simulink subsystem "PvtSubSys_VSM_LCK"  (R2020b)
settings: Solver=VariableStepAuto  StartTime=0.0  StopTime=10.0  RelTol=1e-3
values from neighbouring files (symbols this model uses):
  LCK_STATE : value not decoded    [LCK.sldd]
  P_VSM_LCK_A1 = 15.0    [LCK.sldd]
  P_VSM_LCK_AbsEspInTime = 3.0    [LCK.sldd]
  P_VSM_LCK_absLongitudeAccIn = 2.5    [LCK.sldd]
  P_VSM_LCK_absLongitudeAccOut = 3.0    [LCK.sldd]
  P_VSM_LCK_AccRateIn = 30.0    [LCK.sldd]
  P_VSM_LCK_AccRateInTime = 1.5    [LCK.sldd]
  P_VSM_LCK_AccRateOut = 80.0    [LCK.sldd]
  P_VSM_LCK_AccrPelOut = 30.0    [LCK.sldd]
  P_VSM_LCK_AccrPelRateOut = 0.0    [LCK.sldd]
  P_VSM_LCK_BrakePressIn = 3.0    [LCK.sldd]
  P_VSM_LCK_BrakePressInTime = 1.5    [LCK.sldd]
  P_VSM_LCK_BrakePressOut = 5.0    [LCK.sldd]
  P_VSM_LCK_C0 = 0.4    [LCK.sldd]
  P_VSM_LCK_DrvInputTrqValueIn = 2.0    [LCK.sldd]
  P_VSM_LCK_DrvInputTrqValueInTime = 3.0    [LCK.sldd]
  P_VSM_LCK_DrvInputTrqValueOut = 2.3    [LCK.sldd]
  P_VSM_LCK_dypreFactor = 1.0    [LCK.sldd]
  P_VSM_LCK_IdleInTime = 2.0    [LCK.sldd]
  P_VSM_LCK_LanechangeSwitch = 0.0    [LCK.sldd]
  P_VSM_LCK_LaneDouble = 1.0    [LCK.sldd]
  P_VSM_LCK_Lanewidthswitch = 1.0    [LCK.sldd]
  P_VSM_LCK_LateralAcceIn = 3.0    [LCK.sldd]
  P_VSM_LCK_LateralAcceInTime = 3.0    [LCK.sldd]
  P_VSM_LCK_LateralAcceOut = 3.5    [LCK.sldd]
  P_VSM_LCK_LCDrvInputTrqValueOut = 3.0    [LCK.sldd]
  P_VSM_LCK_LCOverrideTime = 0.6    [LCK.sldd]
  P_VSM_LCK_LCOverrideValue = 1.5    [LCK.sldd]
  P_VSM_LCK_LongitudeAccIn = 3.0    [LCK.sldd]
  P_VSM_LCK_LongitudeAccInTime = 3.0    [LCK.sldd]
  P_VSM_LCK_LongitudeAccOut = 3.5    [LCK.sldd]
  P_VSM_LCK_OverrideInTime = 3.0    [LCK.sldd]
  P_VSM_LCK_OverrideTime = 0.3    [LCK.sldd]
  P_VSM_LCK_OverrideValue = 1.2    [LCK.sldd]
  P_VSM_LCK_ParamA1 : value not decoded    [LCK.sldd]
  P_VSM_LCK_PreTime = 0.2    [LCK.sldd]
  P_VSM_LCK_State_Absesp_enable = 1.0    [LCK.sldd]
  P_VSM_LCK_State_Accpedalrate_enable = 0.0    [LCK.sldd]
  P_VSM_LCK_State_Breakpressure_enable = 1.0    [LCK.sldd]
  P_VSM_LCK_State_DriverInputTrqValue_enable = 1.0    [LCK.sldd]
  P_VSM_LCK_State_Eps_enable = 1.0    [LCK.sldd]
  P_VSM_LCK_State_ESSSts_enable = 1.0    [LCK.sldd]
  P_VSM_LCK_State_GEAR_enable = 1.0    [LCK.sldd]
  P_VSM_LCK_State_Handson_enable = 1.0    [LCK.sldd]
  P_VSM_LCK_State_IdleInTime_enable = 0.0    [LCK.sldd]
  P_VSM_LCK_State_Lane_enable = 1.0    [LCK.sldd]
  P_VSM_LCK_State_LaneChange_enable = 1.0    [LCK.sldd]
  P_VSM_LCK_State_LaneCurve_enable = 0.0    [LCK.sldd]
  P_VSM_LCK_State_LateralAcce_enable = 1.0    [LCK.sldd]
  P_VSM_LCK_State_LongitudeAcc_enable = 1.0    [LCK.sldd]
  P_VSM_LCK_State_LSMLine_enable = 1.0    [LCK.sldd]
  P_VSM_LCK_State_Overide_enable = 1.0    [LCK.sldd]
  P_VSM_LCK_State_Param_LaneCurve : value not decoded    [LCK.sldd]
  P_VSM_LCK_State_Param_LaneCurve_Offset : value not decoded    [LCK.sldd]
  P_VSM_LCK_State_Param_LaneWidth : value not decoded    [LCK.sldd]
  P_VSM_LCK_State_Param_LaneWidth_Offset : value not decoded    [LCK.sldd]
  P_VSM_LCK_State_SteerWheelAngle_enable = 1.0    [LCK.sldd]
  P_VSM_LCK_State_SteerWheelSpd_enable = 1.0    [LCK.sldd]
  P_VSM_LCK_State_TargetLaneIn_enable = 1.0    [LCK.sldd]
  P_VSM_LCK_State_TurnLight_enable = 1.0    [LCK.sldd]
  P_VSM_LCK_State_Vehspeed_enable = 1.0    [LCK.sldd]
  P_VSM_LCK_State_Yawsup_enable = 1.0    [LCK.sldd]
  P_VSM_LCK_SteerAngleSpdIn = 150.0    [LCK.sldd]
  P_VSM_LCK_SteerAngleSpdInTime = 3.0    [LCK.sldd]
  P_VSM_LCK_SteerAngleSpdOut = 200.0    [LCK.sldd]
  P_VSM_LCK_SteerWheelAngleIn = 70.0    [LCK.sldd]
  P_VSM_LCK_SteerWheelAngleInTime = 3.0    [LCK.sldd]
  P_VSM_LCK_SteerWheelAngleOut = 90.0    [LCK.sldd]
  P_VSM_LCK_T0 = 0.75    [LCK.sldd]
  P_VSM_LCK_T1 = 15.0    [LCK.sldd]
  P_VSM_LCK_TargetInSwitch = 0.0    [LCK.sldd]
  P_VSM_LCK_Warnarea1 = -0.55    [LCK.sldd]
  P_VSM_LCK_Warnarea2 = -0.35    [LCK.sldd]
  P_VSM_LCK_YawRateIn = 0.2    [LCK.sldd]
  P_VSM_LCK_YawRateInTime = 1.0    [LCK.sldd]
  P_VSM_LCK_YawRateOut = 0.25    [LCK.sldd]
undefined symbols (not defined in the file or in its folder): P_VSM_LSMC_SampleTime
libraries: simulink x275
(part 4 of 5)

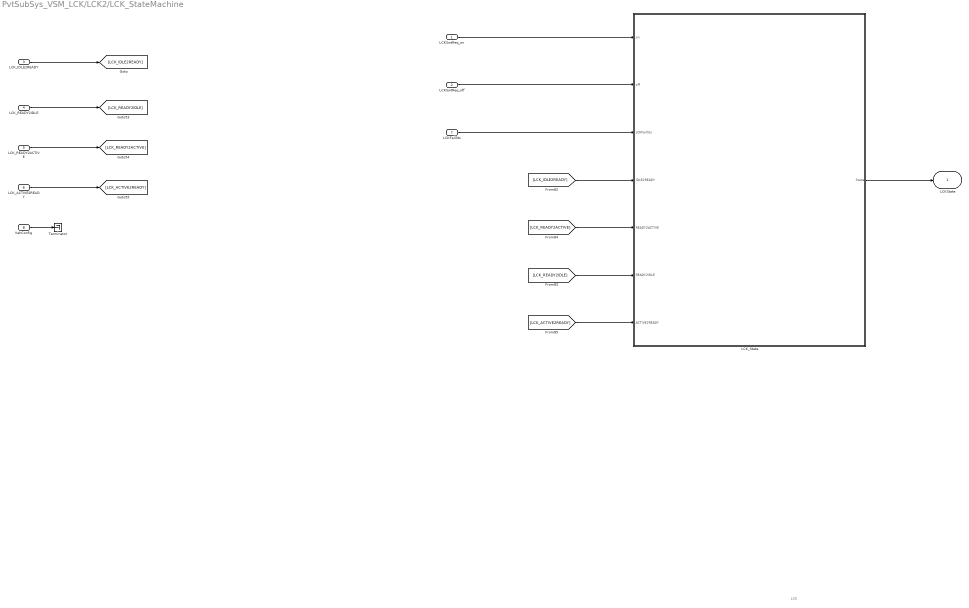
== system PvtSubSys_VSM_LCK/LCK2/LCK_StateMachine ==
  note: LCK
  LCKSwtReq_on : Inport
  LCKSwtReq_off : Inport  Port=2
  LCK_IDLE2READY : Inport  Port=3
  LCK_READY2IDLE : Inport  Port=4
  LCK_READY2ACTIVE : Inport  Port=5
  LCK_ACTIVE2READY : Inport  Port=6
  LCKFailSts : Inport  Port=7
  VehConfig : Inport  Port=8
  LCK_State : Stateflow chart  TreatAsAtomicUnit=on
  Terminator : Terminator
  LCKState : Outport
  wires:
  VehConfig/1 -> Terminator/1
  [LCK_READY2IDLE] -> LCK_State/6(READY2IDLE)
  LCKSwtReq_off/1 -> LCK_State/2(off)
  LCKSwtReq_on/1 -> LCK_State/1(on)
  LCK_ACTIVE2READY/1 -> [LCK_ACTIVE2READY]
  LCK_READY2ACTIVE/1 -> [LCK_READY2ACTIVE]
  LCK_READY2IDLE/1 -> [LCK_READY2IDLE]
  LCK_IDLE2READY/1 -> [LCK_IDLE2READY]
  [LCK_ACTIVE2READY] -> LCK_State/7(ACTIVE2READY)
  LCKFailSts/1 -> LCK_State/3(LCKFailSts)
  LCK_State/1(State) -> LCKState/1
  [LCK_IDLE2READY] -> LCK_State/4(IDLE2READY)
  [LCK_READY2ACTIVE] -> LCK_State/5(READY2ACTIVE)

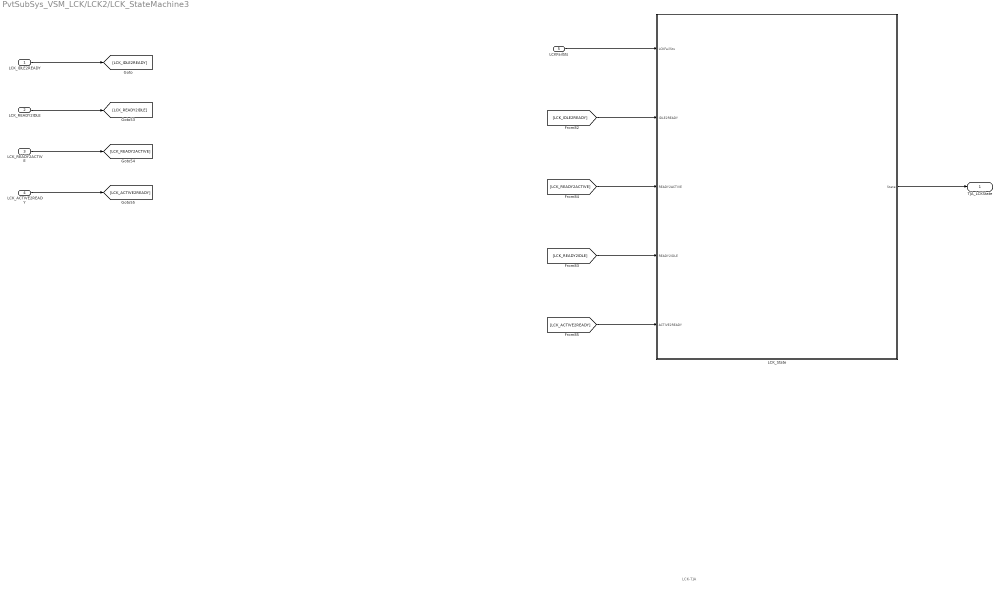
== system PvtSubSys_VSM_LCK/LCK2/LCK_StateMachine3 ==
  note: LCK-TJA
  LCK_IDLE2READY : Inport
  LCK_READY2IDLE : Inport  Port=2
  LCK_READY2ACTIVE : Inport  Port=3
  LCK_ACTIVE2READY : Inport  Port=4
  LCKFailSts : Inport  Port=5
  LCK_State : Stateflow chart  TreatAsAtomicUnit=on
  TJA_LCKState : Outport
  wires:
  [LCK_READY2IDLE] -> LCK_State/4(READY2IDLE)
  LCK_ACTIVE2READY/1 -> [LCK_ACTIVE2READY]
  LCK_READY2ACTIVE/1 -> [LCK_READY2ACTIVE]
  LCK_READY2IDLE/1 -> [LCK_READY2IDLE]
  LCK_IDLE2READY/1 -> [LCK_IDLE2READY]
  [LCK_ACTIVE2READY] -> LCK_State/5(ACTIVE2READY)
  LCKFailSts/1 -> LCK_State/1(LCKFailSts)
  LCK_State/1(State) -> TJA_LCKState/1
  [LCK_IDLE2READY] -> LCK_State/2(IDLE2READY)
  [LCK_READY2ACTIVE] -> LCK_State/3(READY2ACTIVE)

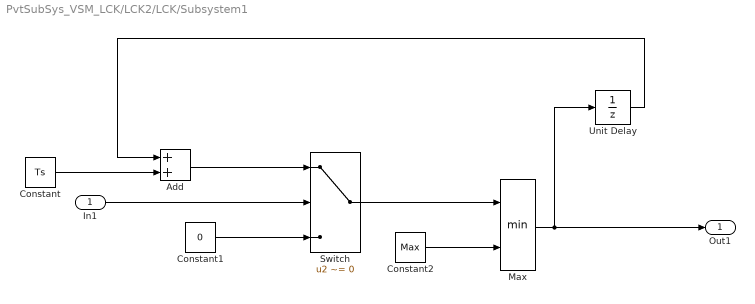
== system PvtSubSys_VSM_LCK/LCK2/LCK/Subsystem1 ==
  In1 : Inport
  Add : Sum
  Constant : Constant  Value=Ts
  Constant1 : Constant  Value=0
  Constant2 : Constant  Value=Max
  Max : MinMax  Inputs=2
  Switch : Switch  Criteria=u2 ~= 0
  Unit Delay : UnitDelay  SampleTime=-1  HasFrameUpgradeWarning=on
  Out1 : Outport
  wires:
  Switch/1 -> Max/1
  Constant2/1 -> Max/2
  Max/1 -> Out1/1, Unit Delay/1
  Add/1 -> Switch/1
  Constant1/1 -> Switch/3
  Constant/1 -> Add/2
  In1/1 -> Switch/2
  Unit Delay/1 -> Add/1

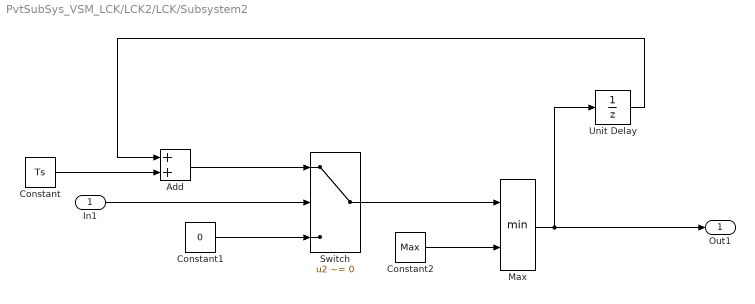
== system PvtSubSys_VSM_LCK/LCK2/LCK/Subsystem2 ==
  In1 : Inport
  Add : Sum
  Constant : Constant  Value=Ts
  Constant1 : Constant  Value=0
  Constant2 : Constant  Value=Max
  Max : MinMax  Inputs=2
  Switch : Switch  Criteria=u2 ~= 0
  Unit Delay : UnitDelay  SampleTime=-1  HasFrameUpgradeWarning=on
  Out1 : Outport
  wires:
  Unit Delay/1 -> Add/1
  In1/1 -> Switch/2
  Constant/1 -> Add/2
  Constant1/1 -> Switch/3
  Add/1 -> Switch/1
  Max/1 -> Unit Delay/1, Out1/1
  Constant2/1 -> Max/2
  Switch/1 -> Max/1

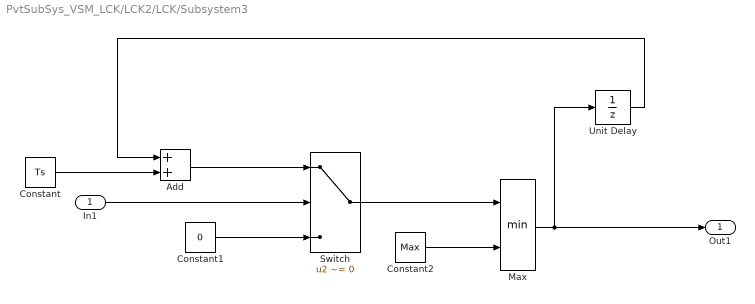
== system PvtSubSys_VSM_LCK/LCK2/LCK/Subsystem3 ==
  In1 : Inport
  Add : Sum
  Constant : Constant  Value=Ts
  Constant1 : Constant  Value=0
  Constant2 : Constant  Value=Max
  Max : MinMax  Inputs=2
  Switch : Switch  Criteria=u2 ~= 0
  Unit Delay : UnitDelay  SampleTime=-1  HasFrameUpgradeWarning=on
  Out1 : Outport
  wires:
  Switch/1 -> Max/1
  Constant2/1 -> Max/2
  Max/1 -> Out1/1, Unit Delay/1
  Add/1 -> Switch/1
  Constant1/1 -> Switch/3
  Constant/1 -> Add/2
  In1/1 -> Switch/2
  Unit Delay/1 -> Add/1

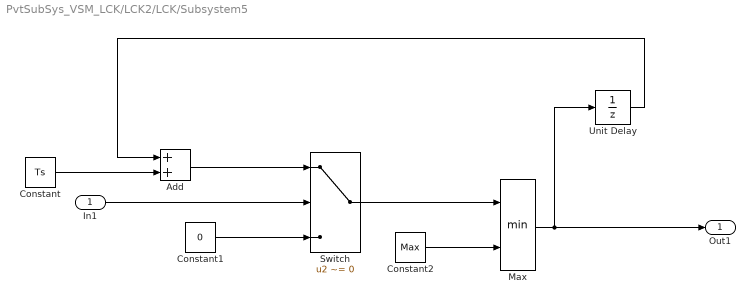
== system PvtSubSys_VSM_LCK/LCK2/LCK/Subsystem5 ==
  In1 : Inport
  Add : Sum
  Constant : Constant  Value=Ts
  Constant1 : Constant  Value=0
  Constant2 : Constant  Value=Max
  Max : MinMax  Inputs=2
  Switch : Switch  Criteria=u2 ~= 0
  Unit Delay : UnitDelay  SampleTime=-1  HasFrameUpgradeWarning=on
  Out1 : Outport
  wires:
  Unit Delay/1 -> Add/1
  In1/1 -> Switch/2
  Constant/1 -> Add/2
  Constant1/1 -> Switch/3
  Add/1 -> Switch/1
  Max/1 -> Unit Delay/1, Out1/1
  Constant2/1 -> Max/2
  Switch/1 -> Max/1

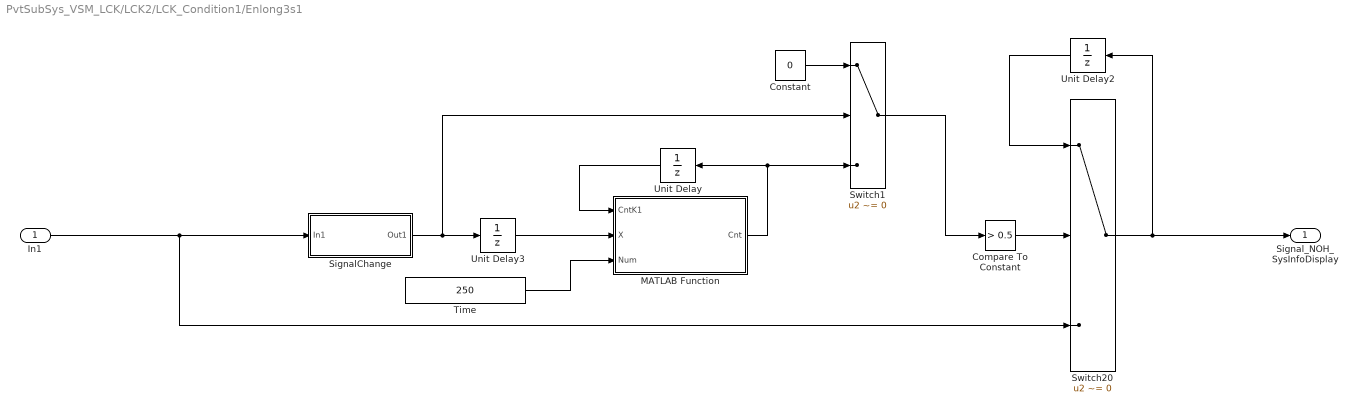
== system PvtSubSys_VSM_LCK/LCK2/LCK_Condition1/Enlong3s1 ==
  In1 : Inport
  Compare To Constant : simulink/Logic and Bit Operations/Compare To Constant  relop=>  const=0.5  OutDataTypeStr=boolean
  Constant : Constant  Value=0  OutDataTypeStr=uint16
  MATLAB Function : MATLAB Function  TreatAsAtomicUnit=on
  SignalChange : Subsystem
  Switch1 : Switch  Criteria=u2 ~= 0
  Switch20 : Switch  Criteria=u2 ~= 0
  Time : Constant  Value=250  OutDataTypeStr=uint16
  Unit Delay : UnitDelay  SampleTime=-1  HasFrameUpgradeWarning=on
  Unit Delay2 : UnitDelay  SampleTime=-1  HasFrameUpgradeWarning=on
  Unit Delay3 : UnitDelay  SampleTime=-1  HasFrameUpgradeWarning=on
  Signal_NOH_SysInfoDisplay : Outport
  wires:
  Time/1 -> MATLAB Function/3(Num)
  Switch20/1 -> Signal_NOH_SysInfoDisplay/1, Unit Delay2/1
  Unit Delay2/1 -> Switch20/1
  Unit Delay3/1 -> MATLAB Function/2(X)
  Compare To Constant/1 -> Switch20/2
  Switch1/1 -> Compare To Constant/1
  MATLAB Function/1(Cnt) -> Unit Delay/1, Switch1/3
  Constant/1 -> Switch1/1
  Unit Delay/1 -> MATLAB Function/1(CntK1)
  SignalChange/1(Out1) -> Unit Delay3/1, Switch1/2
  In1/1 -> SignalChange/1(In1), Switch20/3

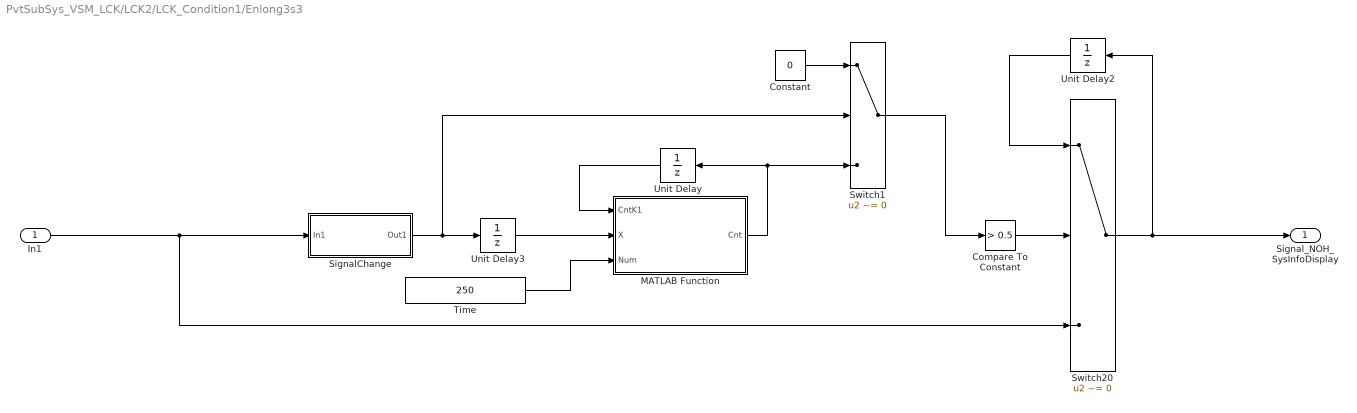
== system PvtSubSys_VSM_LCK/LCK2/LCK_Condition1/Enlong3s3 ==
  In1 : Inport
  Compare To Constant : simulink/Logic and Bit Operations/Compare To Constant  relop=>  const=0.5  OutDataTypeStr=boolean
  Constant : Constant  Value=0  OutDataTypeStr=uint16
  MATLAB Function : MATLAB Function  TreatAsAtomicUnit=on
  SignalChange : Subsystem
  Switch1 : Switch  Criteria=u2 ~= 0
  Switch20 : Switch  Criteria=u2 ~= 0
  Time : Constant  Value=250  OutDataTypeStr=uint16
  Unit Delay : UnitDelay  SampleTime=-1  HasFrameUpgradeWarning=on
  Unit Delay2 : UnitDelay  SampleTime=-1  HasFrameUpgradeWarning=on
  Unit Delay3 : UnitDelay  SampleTime=-1  HasFrameUpgradeWarning=on
  Signal_NOH_SysInfoDisplay : Outport
  wires:
  In1/1 -> Switch20/3, SignalChange/1(In1)
  SignalChange/1(Out1) -> Switch1/2, Unit Delay3/1
  Unit Delay/1 -> MATLAB Function/1(CntK1)
  Constant/1 -> Switch1/1
  MATLAB Function/1(Cnt) -> Switch1/3, Unit Delay/1
  Switch1/1 -> Compare To Constant/1
  Compare To Constant/1 -> Switch20/2
  Unit Delay3/1 -> MATLAB Function/2(X)
  Unit Delay2/1 -> Switch20/1
  Switch20/1 -> Unit Delay2/1, Signal_NOH_SysInfoDisplay/1
  Time/1 -> MATLAB Function/3(Num)

== system PvtSubSys_VSM_LCK/LCK2/LCK_Condition1/Subsystem1 ==
  In1 : Inport
  Add : Sum
  Constant : Constant  Value=Ts
  Constant1 : Constant  Value=0
  Constant2 : Constant  Value=Max
  Max : MinMax  Inputs=2
  Switch : Switch  Criteria=u2 ~= 0
  Unit Delay : UnitDelay  SampleTime=-1  HasFrameUpgradeWarning=on
  Out1 : Outport
  wires:
  Switch/1 -> Max/1
  Constant2/1 -> Max/2
  Max/1 -> Out1/1, Unit Delay/1
  Add/1 -> Switch/1
  Constant1/1 -> Switch/3
  Constant/1 -> Add/2
  In1/1 -> Switch/2
  Unit Delay/1 -> Add/1

== system PvtSubSys_VSM_LCK/LCK2/LCK_Condition1/Subsystem10 ==
  In1 : Inport
  Add : Sum
  Constant : Constant  Value=Ts
  Constant1 : Constant  Value=0
  Constant2 : Constant  Value=Max
  Max : MinMax  Inputs=2
  Switch : Switch  Criteria=u2 ~= 0
  Unit Delay : UnitDelay  SampleTime=-1  HasFrameUpgradeWarning=on
  Out1 : Outport
  wires:
  Unit Delay/1 -> Add/1
  In1/1 -> Switch/2
  Constant/1 -> Add/2
  Constant1/1 -> Switch/3
  Add/1 -> Switch/1
  Max/1 -> Unit Delay/1, Out1/1
  Constant2/1 -> Max/2
  Switch/1 -> Max/1

== system PvtSubSys_VSM_LCK/LCK2/LCK_Condition1/Subsystem11 ==
  In1 : Inport
  Add : Sum
  Constant : Constant  Value=Ts
  Constant1 : Constant  Value=0
  Constant2 : Constant  Value=Max
  Max : MinMax  Inputs=2
  Switch : Switch  Criteria=u2 ~= 0
  Unit Delay : UnitDelay  SampleTime=-1  HasFrameUpgradeWarning=on
  Out1 : Outport
  wires:
  Switch/1 -> Max/1
  Constant2/1 -> Max/2
  Max/1 -> Out1/1, Unit Delay/1
  Add/1 -> Switch/1
  Constant1/1 -> Switch/3
  Constant/1 -> Add/2
  In1/1 -> Switch/2
  Unit Delay/1 -> Add/1

== system PvtSubSys_VSM_LCK/LCK2/LCK_Condition1/Subsystem12 ==
  In1 : Inport
  Add : Sum
  Constant : Constant  Value=Ts
  Constant1 : Constant  Value=0
  Constant2 : Constant  Value=Max
  Max : MinMax  Inputs=2
  Switch : Switch  Criteria=u2 ~= 0
  Unit Delay : UnitDelay  SampleTime=-1  HasFrameUpgradeWarning=on
  Out1 : Outport
  wires:
  Unit Delay/1 -> Add/1
  In1/1 -> Switch/2
  Constant/1 -> Add/2
  Constant1/1 -> Switch/3
  Add/1 -> Switch/1
  Max/1 -> Unit Delay/1, Out1/1
  Constant2/1 -> Max/2
  Switch/1 -> Max/1

== system PvtSubSys_VSM_LCK/LCK2/LCK_Condition1/Subsystem13 ==
  In1 : Inport
  Add : Sum
  Constant : Constant  Value=Ts
  Constant1 : Constant  Value=0
  Constant2 : Constant  Value=Max
  Max : MinMax  Inputs=2
  Switch : Switch  Criteria=u2 ~= 0
  Unit Delay : UnitDelay  SampleTime=-1  HasFrameUpgradeWarning=on
  Out1 : Outport
  wires:
  Switch/1 -> Max/1
  Constant2/1 -> Max/2
  Max/1 -> Out1/1, Unit Delay/1
  Add/1 -> Switch/1
  Constant1/1 -> Switch/3
  Constant/1 -> Add/2
  In1/1 -> Switch/2
  Unit Delay/1 -> Add/1

== system PvtSubSys_VSM_LCK/LCK2/LCK_Condition1/Subsystem14 ==
  In1 : Inport
  Add : Sum
  Constant : Constant  Value=Ts
  Constant1 : Constant  Value=0
  Constant2 : Constant  Value=Max
  Max : MinMax  Inputs=2
  Switch : Switch  Criteria=u2 ~= 0
  Unit Delay : UnitDelay  SampleTime=-1  HasFrameUpgradeWarning=on
  Out1 : Outport
  wires:
  Unit Delay/1 -> Add/1
  In1/1 -> Switch/2
  Constant/1 -> Add/2
  Constant1/1 -> Switch/3
  Add/1 -> Switch/1
  Max/1 -> Unit Delay/1, Out1/1
  Constant2/1 -> Max/2
  Switch/1 -> Max/1

== system PvtSubSys_VSM_LCK/LCK2/LCK_Condition1/Subsystem15 ==
  In1 : Inport
  Add : Sum
  Constant : Constant  Value=Ts
  Constant1 : Constant  Value=0
  Constant2 : Constant  Value=Max
  Max : MinMax  Inputs=2
  Switch : Switch  Criteria=u2 ~= 0
  Unit Delay : UnitDelay  SampleTime=-1  HasFrameUpgradeWarning=on
  Out1 : Outport
  wires:
  Switch/1 -> Max/1
  Constant2/1 -> Max/2
  Max/1 -> Out1/1, Unit Delay/1
  Add/1 -> Switch/1
  Constant1/1 -> Switch/3
  Constant/1 -> Add/2
  In1/1 -> Switch/2
  Unit Delay/1 -> Add/1

== system PvtSubSys_VSM_LCK/LCK2/LCK_Condition1/Subsystem16 ==
  In1 : Inport
  Add : Sum
  Constant : Constant  Value=Ts
  Constant1 : Constant  Value=0
  Constant2 : Constant  Value=Max
  Max : MinMax  Inputs=2
  Switch : Switch  Criteria=u2 ~= 0
  Unit Delay : UnitDelay  SampleTime=-1  HasFrameUpgradeWarning=on
  Out1 : Outport
  wires:
  Unit Delay/1 -> Add/1
  In1/1 -> Switch/2
  Constant/1 -> Add/2
  Constant1/1 -> Switch/3
  Add/1 -> Switch/1
  Max/1 -> Unit Delay/1, Out1/1
  Constant2/1 -> Max/2
  Switch/1 -> Max/1

== system PvtSubSys_VSM_LCK/LCK2/LCK_Condition1/Subsystem17 ==
  In1 : Inport
  Add : Sum
  Constant : Constant  Value=Ts
  Constant1 : Constant  Value=0
  Constant2 : Constant  Value=Max
  Max : MinMax  Inputs=2
  Switch : Switch  Criteria=u2 ~= 0
  Unit Delay : UnitDelay  SampleTime=-1  HasFrameUpgradeWarning=on
  Out1 : Outport
  wires:
  Unit Delay/1 -> Add/1
  In1/1 -> Switch/2
  Constant/1 -> Add/2
  Constant1/1 -> Switch/3
  Add/1 -> Switch/1
  Max/1 -> Unit Delay/1, Out1/1
  Constant2/1 -> Max/2
  Switch/1 -> Max/1

== system PvtSubSys_VSM_LCK/LCK2/LCK_Condition1/Subsystem18 ==
  In1 : Inport
  Add : Sum
  Constant : Constant  Value=Ts
  Constant1 : Constant  Value=0
  Constant2 : Constant  Value=Max
  Max : MinMax  Inputs=2
  Switch : Switch  Criteria=u2 ~= 0
  Unit Delay : UnitDelay  SampleTime=-1  HasFrameUpgradeWarning=on
  Out1 : Outport
  wires:
  Unit Delay/1 -> Add/1
  In1/1 -> Switch/2
  Constant/1 -> Add/2
  Constant1/1 -> Switch/3
  Add/1 -> Switch/1
  Max/1 -> Unit Delay/1, Out1/1
  Constant2/1 -> Max/2
  Switch/1 -> Max/1

== system PvtSubSys_VSM_LCK/LCK2/LCK_Condition1/Subsystem19 ==
  In1 : Inport
  Add : Sum
  Constant : Constant  Value=Ts
  Constant1 : Constant  Value=0
  Constant2 : Constant  Value=Max
  Max : MinMax  Inputs=2
  Switch : Switch  Criteria=u2 ~= 0
  Unit Delay : UnitDelay  SampleTime=-1  HasFrameUpgradeWarning=on
  Out1 : Outport
  wires:
  Switch/1 -> Max/1
  Constant2/1 -> Max/2
  Max/1 -> Out1/1, Unit Delay/1
  Add/1 -> Switch/1
  Constant1/1 -> Switch/3
  Constant/1 -> Add/2
  In1/1 -> Switch/2
  Unit Delay/1 -> Add/1

== system PvtSubSys_VSM_LCK/LCK2/LCK_Condition1/Subsystem2 ==
  In1 : Inport
  Add : Sum
  Constant : Constant  Value=Ts
  Constant1 : Constant  Value=0
  Constant2 : Constant  Value=Max
  Max : MinMax  Inputs=2
  Switch : Switch  Criteria=u2 ~= 0
  Unit Delay : UnitDelay  SampleTime=-1  HasFrameUpgradeWarning=on
  Out1 : Outport
  wires:
  Unit Delay/1 -> Add/1
  In1/1 -> Switch/2
  Constant/1 -> Add/2
  Constant1/1 -> Switch/3
  Add/1 -> Switch/1
  Max/1 -> Unit Delay/1, Out1/1
  Constant2/1 -> Max/2
  Switch/1 -> Max/1

== system PvtSubSys_VSM_LCK/LCK2/LCK_Condition1/Subsystem20 ==
  In1 : Inport
  Add : Sum
  Constant : Constant  Value=Ts
  Constant1 : Constant  Value=0
  Constant2 : Constant  Value=Max
  Max : MinMax  Inputs=2
  Switch : Switch  Criteria=u2 ~= 0
  Unit Delay : UnitDelay  SampleTime=-1  HasFrameUpgradeWarning=on
  Out1 : Outport
  wires:
  Switch/1 -> Max/1
  Constant2/1 -> Max/2
  Max/1 -> Out1/1, Unit Delay/1
  Add/1 -> Switch/1
  Constant1/1 -> Switch/3
  Constant/1 -> Add/2
  In1/1 -> Switch/2
  Unit Delay/1 -> Add/1

== system PvtSubSys_VSM_LCK/LCK2/LCK_Condition1/Subsystem21 ==
  In1 : Inport
  Add : Sum
  Constant : Constant  Value=Ts
  Constant1 : Constant  Value=0
  Constant2 : Constant  Value=Max
  Max : MinMax  Inputs=2
  Switch : Switch  Criteria=u2 ~= 0
  Unit Delay : UnitDelay  SampleTime=-1  HasFrameUpgradeWarning=on
  Out1 : Outport
  wires:
  Switch/1 -> Max/1
  Constant2/1 -> Max/2
  Max/1 -> Out1/1, Unit Delay/1
  Add/1 -> Switch/1
  Constant1/1 -> Switch/3
  Constant/1 -> Add/2
  In1/1 -> Switch/2
  Unit Delay/1 -> Add/1

== system PvtSubSys_VSM_LCK/LCK2/LCK_Condition1/Subsystem3 ==
  In1 : Inport
  Add : Sum
  Constant : Constant  Value=Ts
  Constant1 : Constant  Value=0
  Constant2 : Constant  Value=Max
  Max : MinMax  Inputs=2
  Switch : Switch  Criteria=u2 ~= 0
  Unit Delay : UnitDelay  SampleTime=-1  HasFrameUpgradeWarning=on
  Out1 : Outport
  wires:
  Unit Delay/1 -> Add/1
  In1/1 -> Switch/2
  Constant/1 -> Add/2
  Constant1/1 -> Switch/3
  Add/1 -> Switch/1
  Max/1 -> Unit Delay/1, Out1/1
  Constant2/1 -> Max/2
  Switch/1 -> Max/1

== system PvtSubSys_VSM_LCK/LCK2/LCK_Condition1/Subsystem4 ==
  In1 : Inport
  Add : Sum
  Constant : Constant  Value=Ts
  Constant1 : Constant  Value=0
  Constant2 : Constant  Value=Max
  Max : MinMax  Inputs=2
  Switch : Switch  Criteria=u2 ~= 0
  Unit Delay : UnitDelay  SampleTime=-1  HasFrameUpgradeWarning=on
  Out1 : Outport
  wires:
  Unit Delay/1 -> Add/1
  In1/1 -> Switch/2
  Constant/1 -> Add/2
  Constant1/1 -> Switch/3
  Add/1 -> Switch/1
  Max/1 -> Unit Delay/1, Out1/1
  Constant2/1 -> Max/2
  Switch/1 -> Max/1

== system PvtSubSys_VSM_LCK/LCK2/LCK_Condition1/Subsystem5 ==
  In1 : Inport
  Add : Sum
  Constant : Constant  Value=Ts
  Constant1 : Constant  Value=0
  Constant2 : Constant  Value=Max
  Max : MinMax  Inputs=2
  Switch : Switch  Criteria=u2 ~= 0
  Unit Delay : UnitDelay  SampleTime=-1  HasFrameUpgradeWarning=on
  Out1 : Outport
  wires:
  Switch/1 -> Max/1
  Constant2/1 -> Max/2
  Max/1 -> Out1/1, Unit Delay/1
  Add/1 -> Switch/1
  Constant1/1 -> Switch/3
  Constant/1 -> Add/2
  In1/1 -> Switch/2
  Unit Delay/1 -> Add/1

== system PvtSubSys_VSM_LCK/LCK2/LCK_Condition1/Subsystem7 ==
  In1 : Inport
  Add : Sum
  Constant : Constant  Value=Ts
  Constant1 : Constant  Value=0
  Constant2 : Constant  Value=Max
  Max : MinMax  Inputs=2
  Switch : Switch  Criteria=u2 ~= 0
  Unit Delay : UnitDelay  SampleTime=-1  HasFrameUpgradeWarning=on
  Out1 : Outport
  wires:
  Switch/1 -> Max/1
  Constant2/1 -> Max/2
  Max/1 -> Out1/1, Unit Delay/1
  Add/1 -> Switch/1
  Constant1/1 -> Switch/3
  Constant/1 -> Add/2
  In1/1 -> Switch/2
  Unit Delay/1 -> Add/1

== system PvtSubSys_VSM_LCK/LCK2/LCK_Condition1/Subsystem8 ==
  In1 : Inport
  Add : Sum
  Constant : Constant  Value=Ts
  Constant1 : Constant  Value=0
  Constant2 : Constant  Value=Max
  Max : MinMax  Inputs=2
  Switch : Switch  Criteria=u2 ~= 0
  Unit Delay : UnitDelay  SampleTime=-1  HasFrameUpgradeWarning=on
  Out1 : Outport
  wires:
  Switch/1 -> Max/1
  Constant2/1 -> Max/2
  Max/1 -> Out1/1, Unit Delay/1
  Add/1 -> Switch/1
  Constant1/1 -> Switch/3
  Constant/1 -> Add/2
  In1/1 -> Switch/2
  Unit Delay/1 -> Add/1

== system PvtSubSys_VSM_LCK/LCK2/LCK_Condition1/Subsystem9 ==
  In1 : Inport
  Add : Sum
  Constant : Constant  Value=Ts
  Constant1 : Constant  Value=0
  Constant2 : Constant  Value=Max
  Max : MinMax  Inputs=2
  Switch : Switch  Criteria=u2 ~= 0
  Unit Delay : UnitDelay  SampleTime=-1  HasFrameUpgradeWarning=on
  Out1 : Outport
  wires:
  Unit Delay/1 -> Add/1
  In1/1 -> Switch/2
  Constant/1 -> Add/2
  Constant1/1 -> Switch/3
  Add/1 -> Switch/1
  Max/1 -> Unit Delay/1, Out1/1
  Constant2/1 -> Max/2
  Switch/1 -> Max/1

== system PvtSubSys_VSM_LCK/LCK2/LCK_Condition1/Enlong3s1/SignalChange ==
  In1 : Inport
  Compare To Constant1 : simulink/Logic and Bit Operations/Compare To Constant  relop=~=  const=0  OutDataTypeStr=boolean
  Detect Decrease : simulink/Logic and Bit Operations/Detect Decrease  vinit=0.0  OutDataTypeStr=boolean
  Detect Increase3 : simulink/Logic and Bit Operations/Detect Increase  vinit=0.0  OutDataTypeStr=boolean
  Logical Operator : Logic  Operator=OR  AllPortsSameDT=off  OutDataTypeStr=boolean
  Logical Operator1 : Logic  AllPortsSameDT=off  OutDataTypeStr=boolean
  Out1 : Outport
  wires:
  Detect Decrease/1 -> Logical Operator/1
  Logical Operator/1 -> Logical Operator1/2
  Logical Operator1/1 -> Out1/1
  Compare To Constant1/1 -> Logical Operator1/1
  Detect Increase3/1 -> Logical Operator/2
  In1/1 -> Compare To Constant1/1, Detect Decrease/1, Detect Increase3/1

== system PvtSubSys_VSM_LCK/LCK2/LCK_Condition1/Enlong3s3/SignalChange ==
  In1 : Inport
  Compare To Constant1 : simulink/Logic and Bit Operations/Compare To Constant  relop=~=  const=0  OutDataTypeStr=boolean
  Detect Decrease : simulink/Logic and Bit Operations/Detect Decrease  vinit=0.0  OutDataTypeStr=boolean
  Detect Increase3 : simulink/Logic and Bit Operations/Detect Increase  vinit=0.0  OutDataTypeStr=boolean
  Logical Operator : Logic  Operator=OR  AllPortsSameDT=off  OutDataTypeStr=boolean
  Logical Operator1 : Logic  AllPortsSameDT=off  OutDataTypeStr=boolean
  Out1 : Outport
  wires:
  In1/1 -> Detect Increase3/1, Detect Decrease/1, Compare To Constant1/1
  Detect Increase3/1 -> Logical Operator/2
  Compare To Constant1/1 -> Logical Operator1/1
  Logical Operator1/1 -> Out1/1
  Logical Operator/1 -> Logical Operator1/2
  Detect Decrease/1 -> Logical Operator/1

== matlab function PvtSubSys_VSM_LCK/LCK2/LCK/MATLAB Function2 ==
  data: OutCount input single size=1; InCount input single size=1; LCK_LeftWarn input boolean size=1; LCKWarning output uint8 size=1; LCK_RightWarn input boolean size=1; LCKState input uint8 size=1; LCKWarningK1 input uint8 size=1
function LCKWarning = fcn(OutCount, InCount, LCK_LeftWarn, LCK_RightWarn, LCKState, LCKWarningK1)
LCKWarning=uint8(0);
if LCKWarningK1==uint8(3)       %default状态
    if LCK_LeftWarn==uint8(1) && LCKState==uint8(3) && InCount>single(150) %抑制3s
        LCKWarning=uint8(1);
    elseif LCK_RightWarn==uint8(1) && LCKState==uint8(3) && InCount>single(150)
        LCKWarning=uint8(2);
    elseif LCK_LeftWarn==uint8(0) && LCK_RightWarn==uint8(0)
        LCKWarning=uint8(0);
    else
        LCKWarning=uint8(3);
    end
elseif  LCKWarningK1==uint8(1) || LCKWarningK1==uint8(2)   %非default状态
    if LCK_LeftWarn==uint8(1) && LCK_RightWarn==uint8(0) && LCKState==uint8(3)
        if OutCount<single(200)  %4s后抑制
            LCKWarning=uint8(1);
        else
            LCKWarning=uint8(3);
        end
    elseif LCK_LeftWarn==uint8(0) && LCK_RightWarn==uint8(1) && LCKState==uint8(3)
        if OutCount<single(200)
            LCKWarning=uint8(2);
        else
            LCKWarning=uint8(3);
        end
        
    elseif LCK_LeftWarn==uint8(0) && LCK_RightWarn==uint8(0)
        LCKWarning=uint8(0);
    end
elseif  LCKWarningK1==uint8(0)
    if LCK_LeftWarn==uint8(1) && LCK_RightWarn==uint8(0) && LCKState==uint8(3)
        LCKWarning=uint8(1);
    elseif LCK_LeftWarn==uint8(0) && LCK_RightWarn==uint8(1) && LCKState==uint8(3)
        LCKWarning=uint8(2);
    end
end

== matlab function PvtSubSys_VSM_LCK/LCK2/LCK/MATLAB Function3 ==
  data: data input single size=1; LCKWarning input uint8 size=1; OutCount output single size=1; InCount output single size=1; data1 input single size=1
function [OutCount,InCount] = fcn(data, LCKWarning, data1)
OutCount=single(0);
 InCount=single(0);
if LCKWarning==uint8(1) || LCKWarning==uint8(2)
    OutCount=data+1;  
elseif LCKWarning==uint8(3)
    InCount=data1+1;
end

== matlab function PvtSubSys_VSM_LCK/LCK2/LCK_Condition1/MATLAB Function ==
  data: LeftChangefg input; y output; RightChangefg input; Ldy input; Rdy input; Lfgk1 input; Lfg output; Rfgk1 input; Rfg output
function [y,Lfg,Rfg] = fcn(LeftChangefg,RightChangefg,Ldy,Rdy,Lfgk1,Rfgk1)
y=1;
Lfg=0;
Rfg=0;
if LeftChangefg>0
    Lfg=1;
    y=0;
elseif Lfgk1>0
    Lfg=1;
    y=0;
    if Rdy>0
        Lfg=0;
        y=1;
    end
    
end

if RightChangefg>0
    Rfg=1;
    y=0;
elseif Rfgk1>0
    Rfg=1;
    y=0;
    if Ldy>0
        Rfg=0;
        y=1;
    end
    
end

== matlab function PvtSubSys_VSM_LCK/LCK2/LCK_Condition1/MATLAB Function3 ==
  data: Ready2Idle input; Ready2IdleK1 input; LCKSts input; CountK1 input; Count output
function Count= fcn(Ready2Idle,Ready2IdleK1,LCKSts,CountK1)
Count=0;
if LCKSts==1
    if Ready2Idle==1 || Ready2IdleK1==1
        Count=CountK1+1;
    elseif CountK1>0 && Ready2Idle==0
        Count=CountK1+1;
    end
elseif LCKSts==2 || LCKSts==3 
    Count=0;
elseif LCKSts==0 || LCKSts==7
    Count=9999;
end

== stateflow chart PvtSubSys_VSM_LCK/LCK2/LCK_StateMachine/LCK_State ==
  state MAINST_ERROR
    en:State=LCK_STATE.LCK_Error;
  state MAINST_OFF
    en:State=LCK_STATE.LCK_Off;
  state MAINST_ON
    state SUBST_IDLE
      en: State=LCK_STATE.LCK_Idle;
    state enabled
      state SUBST_READY
        en:State=LCK_STATE.LCK_Ready;
      state SUBST_ACTIVE
        en:State=LCK_STATE.LCK_Active;
      (default) -> (junction 367)
      (junction 367) -> SUBST_READY [order 2]
      (junction 367) -> SUBST_ACTIVE [order 1] : [READY2ACTIVE]
      SUBST_READY -> SUBST_ACTIVE : [READY2ACTIVE]
      SUBST_ACTIVE -> SUBST_READY : [ACTIVE2READY]
    (junction 366) -> SUBST_IDLE [order 2]
    SUBST_IDLE -> enabled : [IDLE2READY]
    enabled -> SUBST_IDLE : [READY2IDLE]
    (default) -> (junction 366)
    (junction 366) -> enabled [order 1] : [IDLE2READY]
  (default) -> MAINST_OFF
  MAINST_OFF -> MAINST_ERROR [order 1] : [LCKFailSts==1 && on ]
  MAINST_ERROR -> MAINST_OFF [order 1] : [off]
  MAINST_OFF -> MAINST_ON [order 2] : [on]
  MAINST_ON -> MAINST_OFF [order 1] : [off]
  MAINST_ON -> MAINST_ERROR [order 2] : [LCKFailSts==1]
  MAINST_ERROR -> MAINST_ON [order 2] : [LCKFailSts==0]
  data: on input; off input; LCKFailSts input; State output Enum: LCK_STATE =LCK_STATE.LCK_Off;; IDLE2READY input; READY2ACTIVE input; READY2IDLE input; ACTIVE2READY input
